simulink model "randomVelToLeader"  (R2016a)
settings: Solver=FixedStepAuto  StartTime=0.0  StopTime=inf  RelTol=1e-3
undefined symbols (not defined in the file or in its folder): Angular, Linear
libraries: robotlib x2, simulink x1
settings Model: Creator=ece446  LastModifiedBy=ece446
settings OptimizationCC: OptimizeModelRefInitCode=on  LifeSpan=Inf  MaxStackSize=64
settings HardwareCC: ProdBitPerPointer=32  ProdLargestAtomicFloat=None  ProdIntDivRoundTo=Undefined  ProdEndianess=Unspecified  ProdWordSize=32  ProdHWDeviceType=Generic->Unspecified (assume 32-bit Generic)  UseEmbeddedCoderFeatures=off
settings RTWCC: SystemTargetFile=ert.tlc  HardwareBoard=Robot Operating System (ROS)  TemplateMakefile=ert_default_tmf  GenerateReport=on  Toolchain=Catkin  IncludeHyperlinkInReport=on  LaunchReport=on  TargetLang=C++  GenerateTraceInfo=on  GenerateTraceReport=on  GenerateTraceReportSl=on  GenerateTraceReportSf=on  GenerateTraceReportEml=on
settings CodeAppCC: ForceParamTrailComments=on  IgnoreCustomStorageClasses=off  OperatorAnnotations=on  SimulinkDataObjDesc=on  SFDataObjDesc=on  MATLABFcnDesc=on  InsertBlockDesc=on  MATLABSourceComments=on
settings ERTTargetCC: SupportNonInlinedSFcns=on

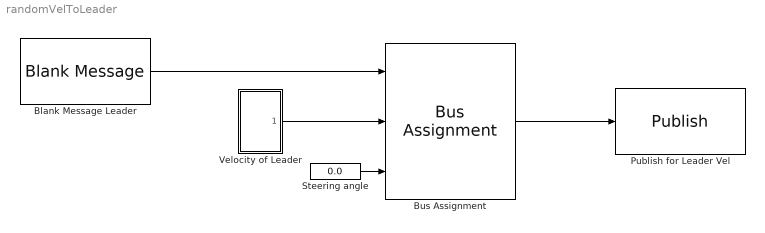
== system randomVelToLeader ==
  Blank Message Leader : robotlib/Blank Message  SourceLibraryInfo=This block requires Robotics System Toolbox  messageType=geometry_msgs/Twist  SampleTime=inf
  Bus Assignment : BusAssignment  AssignedSignals=Linear.X,Angular.Z
  Publish for Leader Vel : robotlib/Publish  SourceLibraryInfo=This block requires Robotics System Toolbox  topicSource=Select from ROS network  topic=/azcar_sim/cmd_vel  messageType=geometry_msgs/Twist  messageQueueLength=1
  Steering angle : Constant  Value=0.0
  Velocity of Leader : Subsystem
  wires:
  Blank Message Leader/1 -> Bus Assignment/1
  Bus Assignment/1 -> Publish for Leader Vel/1
  Velocity of Leader/1(Velocity) -> Bus Assignment/2
  Steering angle/1 -> Bus Assignment/3

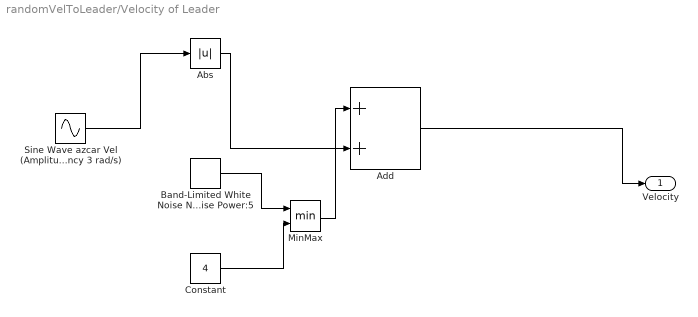
== system randomVelToLeader/Velocity of Leader ==
  Abs : Abs
  Add : Sum
  Band-Limited White Noise Noise Power:5 : simulink/Sources/Band-Limited White Noise  Cov=5  Ts=0.1  seed=[5]
  Constant : Constant  Value=4
  MinMax : MinMax  Inputs=2
  "Sine Wave azcar Vel (Amplitude 5, Frequency 3 rad/s)" : Sin  Amplitude=5  Frequency=3  SampleTime=0
  Velocity : Outport
  wires:
  "Sine Wave azcar Vel (Amplitude 5, Frequency 3 rad/s)"/1 -> Abs/1
  Band-Limited White Noise Noise Power:5/1 -> MinMax/1
  Abs/1 -> Add/2
  Constant/1 -> MinMax/2
  MinMax/1 -> Add/1
  Add/1 -> Velocity/1
